simulink model "TV_FLC_codegen"  (R2025b)
settings: Solver=FixedStepDiscrete  StartTime=0.0  StopTime=100  FixedStep=0.003  MaxStep=0.4  RelTol=1e-3  AbsTol=1e-3
PreLoadFcn:
  | % Due to usability issue in Repeating Sequence block
  | warning('off','Simulink:Masking:Invalid');
  | 
  | % Eliminate unnecessary warnings in inactive variants
  | % Warnings generated only if you click through inactive variant
  | warning('off','MATLAB:nonExistentField');
  | warning('off','Simulink:Parameters:BlkParamUndefined');
PostLoadFcn:
  | set_param([bdroot '/Vehicle'],'popup_trailer','Off')
  | warning('off','sm:sli:setup:compile:LocalSolverNotSupported')
  | %sm_car_config_maneuver(bdroot,'WOT Braking');
  | sm_car_config_vehicle(bdroot,'false');
  | sm_car_config_logging(bdroot);
InitFcn:
  | sm_car_config_camera;
  | Vehicle = sm_car_vehcfg_checkConfig(Vehicle);
  | sm_car_check_tire_model(bdroot);
StartFcn:
  | tic;
StopFcn:
  | Elapsed_Sim_Time = toc;
  | % disp(['Elapsed Sim Time = ' num2str(Elapsed_Sim_Time)]);
model workspace (MAT data in the model file):
  Af = 1.20000004768
  C_alpha_F = 46504
  Control : object (value not decoded)
  F = 0.0421790704131
  FIS_1 : mamfis (value not decoded)
  FIS_2 : mamfis (value not decoded)
  FIS_3 : fistree (value not decoded)
  Gr = 5
  Ku = -0.000124337399029
  L = 1.57799994946
  Load_Ref = [0; 400; 500; 600; 700; 800; 900; 1000; 1100; 1200; 1300; 1400; 1500; 1600; 1700; 1800; 1900; 2000]
  MotorT = [51.0306892395 51.0306892395 51.0306892395 51.0306892395 51.0306892395 51.0306892395 51.0306892395 51.0306892395 51.0306892395 51.0306892395 51.0306892395 51.0306892395 51.0306892395 51.0306892395 51.0306892395 51.0306892395 51.0306892395 51.0306892395 51.0306892395 51.0306892395 51.0306892395 51.0306892395 51.0306892395 51.0306892395 51.0306892395 51.0306892395 51.0306892395 51.0306892395 51.0306892395 51.0306892395 51.0306892395 51.0306892395 51.0306892395 51.0306892395 51.0306892395 51.0306892395 51.0306892395 44.8436889648 36.8215675354 30.0627288818 25.3370742798 21.0374126434 17.0840320587 13.4184885025 9.99592685699 6.7769651413 3.73957490921]
  MotorW = [0 100 200 300 400 500 600 700 800 900 1000 1100 1200 1300 1400 1500 1600 1700 1800 1900 2000 2100 2200 2300 2400 2500 2600 2700 2800 2900 3000 3100 3200 3300 3400 3500 3600 3700 3800 3900 4000 4100 4200 4300 4400 4500 4600]
  Slip_Ctrl_Kd = Simulink.Parameter
  Slip_Ctrl_Kd.Value = 11
  Slip_Ctrl_Kd.Complexity = 'real'
  Slip_Ctrl_Kd.Dimensions = [1 1]
  Slip_Ctrl_Kd.CoderInfo.StorageClass = 'ImportedExtern'
  Slip_Ctrl_Kd.DataType = 'single'
  Slip_Ctrl_Ki = Simulink.Parameter
  Slip_Ctrl_Ki.Value = 6000
  Slip_Ctrl_Ki.Complexity = 'real'
  Slip_Ctrl_Ki.Dimensions = [1 1]
  Slip_Ctrl_Ki.CoderInfo.StorageClass = 'ImportedExtern'
  Slip_Ctrl_Ki.DataType = 'single'
  Slip_Ctrl_Kn = Simulink.Parameter
  Slip_Ctrl_Kn.Value = 100
  Slip_Ctrl_Kn.Complexity = 'real'
  Slip_Ctrl_Kn.Dimensions = [1 1]
  Slip_Ctrl_Kn.CoderInfo.StorageClass = 'ImportedExtern'
  Slip_Ctrl_Kn.DataType = 'single'
  Slip_Ctrl_Kp = Simulink.Parameter
  Slip_Ctrl_Kp.Value = 800
  Slip_Ctrl_Kp.Complexity = 'real'
  Slip_Ctrl_Kp.Dimensions = [1 1]
  Slip_Ctrl_Kp.CoderInfo.StorageClass = 'ImportedExtern'
  Slip_Ctrl_Kp.DataType = 'single'
  Slip_Ref = [0.0799999982119; 0.0799999982119; 0.0900000035763; 0.0949999988079; 0.0930000022054; 0.0920000001788; 0.0909999981523; 0.0900000035763; 0.0900000035763; 0.0900000035763; 0.0939999967813; 0.097999997437; 0.104000002146; 0.112000003457; 0.126000002027; 0.153999999166; 0.20000000298; 0.119999997318]
  Tmax = 51.0306892395
  a = 0.823199987411
  a_cop = 0.707000017166
  cd = -2.15000009537
  g = 9.81000041962
  h_CG = 0.358300000429
  m = 320
  ro = 1.22599995136
  rwheel = 0.263000011444
  steerRatio = 0.175131350756
  tr = 1.24800002575
  vx_th = 0.699999988079
libraries: simulink x5, fuzblock x3, slpidlib x2
(part 1 of 2)
settings Model: Creator=smiller  LastModifiedBy=andrei
settings SolverCC: MaxConsecutiveMinStep=5  AlgebraicLoopSolver=TrustRegion  AutoInsertRateTranBlk=on  InsertRTBMode=Never (minimum delay)  MinimalZcImpactIntegration=on
settings DataIOCC: MaxDataPoints=10000  SaveFormat=StructureWithTime  SaveOutput=off  SignalLogging=off  DSMLogging=off  SaveTime=off  ReturnWorkspaceOutputs=off  SignalLoggingName=logsout_sm_car
settings OptimizationCC: DefaultParameterBehavior=Inlined  UseDivisionForNetSlopeComputation=on  GainParamInheritBuiltInType=on  UseFloatMulNetSlope=on  DefaultUnderspecifiedDataType=single  UseSpecifiedMinMax=on  PassReuseOutputArgsAs=Individual arguments  NoFixptDivByZeroProtection=on  EfficientFloat2IntCast=on  LifeSpan=inf  OptimizeBlockOrder=speed  DifferentSizesBufferReuse=on  EfficientTunableParamExpr=on
settings DebuggingCC: ReadBeforeWriteMsg=EnableAllAsError  WriteAfterWriteMsg=EnableAllAsError  WriteAfterReadMsg=EnableAllAsError  AlgebraicLoopMsg=none  IntegerOverflowMsg=error  ParameterPrecisionLossMsg=none  ParameterTunabilityLossMsg=error  UnconnectedInputMsg=warning  UnconnectedOutputMsg=warning  UnconnectedLineMsg=warning  UniqueDataStoreMsg=error  NonBusSignalsTreatedAsBus=error  SFInvalidInputDataAccessInChartInitDiag=error  SFTransitionOutsideNaturalParentDiag=error  SFUnreachableExecutionPathDiag=error  SFUndirectedBroadcastEventsDiag=error  IntegerSaturationMsg=error  ArithmeticOperatorsInVariantConditions=warning
settings HardwareCC: ProdBitPerPointer=32.0  ProdBitPerSizeT=32.0  ProdBitPerPtrDiffT=32.0  ProdLargestAtomicInteger=Long  ProdLargestAtomicFloat=Double  ProdWordSize=32.0  ProdHWDeviceType=ARM Compatible->ARM Cortex-M
settings ModelReferenceCC: EnableRefExpFcnMdlSchedulingChecks=on
settings SFSimCC: MATLABDynamicMemAlloc=off  CustomCodeUndefinedFunction=UseInterfaceOnly
settings RTWCC: SystemTargetFile=ert.tlc  TemplateMakefile=ert_default_tmf  BuildConfiguration=Faster Runs  GPUComputeCapability=3.5  DLArmComputeVersion=19.05  Description=Embedded Coder
settings CodeAppCC: ForceParamTrailComments=on  IgnoreCustomStorageClasses=off  OperatorAnnotations=on  SimulinkDataObjDesc=on  SFDataObjDesc=on  CustomSymbolStrGlobalVar=rt$N_$R$M  CustomSymbolStrType=$N_$R$M  CustomSymbolStrFcn=$N$M$F  CustomSymbolStrMacro=$N$M  CustomSymbolStrUtil=$N_$R$C  InsertBlockDesc=on
settings ERTTargetCC: ERTCustomFileTemplate=example_file_process.tlc  ERTFilePackagingFormat=CompactWithDataFile  GenerateSampleERTMain=on  IncludeMdlTerminateFcn=off  CombineSignalStateStructs=on  SuppressErrorStatus=on  SupportAbsoluteTime=off  CodeInterfacePackaging=Reusable function  SupportComplex=off
settings SimscapeCC: SimscapeLogType=all  SimscapeLogSimulationStatistics=on  SimscapeLogName=simlog_sm_car  SimscapeLogDataHistory=100000.0  SimscapeOperatingPoint=ssc_op
settings DiagnosticsConfigSet: SimMechanicsConflictingReferenceFrames=none  SimMechanicsRigidlyBoundBlock=none  SimMechanicsUnsatisfiedHighPriorityTargets=error
settings ExplorerConfigSet: InternalSimMechanicsExplorerSettings="<ExplorerConfiguration><canonicalview>default</canonicalview><AnimationSetting><BasePlaybackSpeed>1.0</BasePlaybackSpeed><PlaybackSpeedFactor>1.0</PlaybackSpeedFactor></AnimationSetting><TilePanel><TileInfo><Tiles Columns=\"1\" Count=\"1\" Rows=\"1\"><Column Weight=\"1\"/><Row Weight=\"1\"/><Tile Height=\"1\" Width=\"1\" X=\"0\" Y=\"0\"/></Tiles></TileInfo><SceneInfo><SceneViewer><BGColor><R>1</R><G>1</G><B>1</B></BGColor><Camera><DoPerspective>on</DoPerspective><Position><X>-22.5734563329168161</X><Y>-2.56079992530625722</Y><Z>1.4393604008155032</Z></Position><Center><X>-23.2962680852000119</X><Y>-1.95845679840359432</Y><Z>1.10064823948317181</Z></Center><Up><X>-0.260205889993916473</X><Y>0.216838241661597014</Y><Z>0.940890042335224552</Z></Up><ViewLimDist>1</ViewLimDist><YLim>0.466307658154998694</YLim><XLim>0.489818968650208741</XLim></Camera></SceneViewer></SceneInfo></TilePanel><MechEditorPanel><Cameras><Camera><Id>Camera1</Id><Value><Name>Track FixO FR</Name><NativeCamera><PositionTrackingFeature>Camera_Frames.Frame_FixO_FR.R</PositionTrackingFeature><CenterTrackingFeature>Camera_Frames.Frame_FixO_FR.R</CenterTrackingFeature><UpVectorTrackingFeature>Camera_Frames.Frame_FixO_FR.R</UpVectorTrackingFeature><CenterTrackingOrigin>off</CenterTrackingOrigin><CenterTrackingDirection>+X</CenterTrackingDirection><UpVectorTrackingDirection>+Z</UpVectorTrackingDirection></NativeCamera></Value></Camera><Camera><Id>Camera2</Id><Value><Name>Track FixO Right</Name><NativeCamera><PositionTrackingFeature>Camera_Frames.Frame_FixO_Right.R</PositionTrackingFeature><CenterTrackingFeature>Camera_Frames.Transform_Camera_Ref.F</CenterTrackingFeature><UpVectorTrackingFeature>Camera_Frames.Frame_FixO_Right.R</UpVectorTrackingFeature><CenterTrackingOrigin>off</CenterTrackingOrigin><CenterTrackingDirection>+Y</CenterTrackingDirection><UpVectorTrackingDirection>+Z</UpVectorTrackingDirection></NativeCamera></Value></Camera><Camera><Id>Camera3</Id><Value><Name>Track FixO RR</Name><NativeCamera><PositionTrackingFeature>Camera_Frames.Frame_FixO_RR.R</PositionTrackingFeature><CenterTrackingFeature>Camera_Frames.Frame_FixO_RR.R</CenterTrackingFeature><UpVectorTrackingFeature>Camera_Frames.Frame_FixO_RR.R</UpVectorTrackingFeature><CenterTrackingOrigin>off</CenterTrackingOrigin><CenterTrackingDirection>+X</CenterTrackingDirection><UpVectorTrackingDirection>+Z</UpVectorTrackingDirection></NativeCamera></Value></Camera><Camera><Id>Camera4</Id><Value><Name>Track FixO RL</Name><NativeCamera><PositionTrackingFeature>Camera_Frames.Frame_FixO_RL.R</PositionTrackingFeature><CenterTrackingFeature>Camera_Frames.Frame_FixO_RL.R</CenterTrackingFeature><UpVectorTrackingFeature>Camera_Frames.Frame_FixO_RL.R</UpVectorTrackingFeature><CenterTrackingOrigin>off</CenterTrackingOrigin><CenterTrackingDirection>+X</CenterTrackingDirection><UpVectorTrackingDirection>+Z</UpVectorTrackingDirection></NativeCamera></Value></Camera><Camera><Id>Camera5</Id><Value><Name>Track FixO Left</Name><NativeCamera><PositionTrackingFeature>Camera_Frames.Frame_FixO_Left.R</PositionTrackingFeature><CenterTrackingFeature>Camera_Frames.Transform_Camera_Ref.F</CenterTrackingFeature><UpVectorTrackingFeature>Camera_Frames.Frame_FixO_Left.R</UpVectorTrackingFeature><CenterTrackingOrigin>off</CenterTrackingOrigin><CenterTrackingDirection>-Y</CenterTrackingDirection><UpVectorTrackingDirection>+Z</UpVectorTrackingDirection></NativeCamera></Value></Camera><Camera><Id>Camera6</Id><Value><Name>Track FixO FL</Name><NativeCamera><PositionTrackingFeature>Camera_Frames.Frame_FixO_FL.R</PositionTrackingFeature><CenterTrackingFeature>Camera_Frames.Frame_FixO_FL.R</CenterTrackingFeature><UpVectorTrackingFeature>Camera_Frames.Frame_FixO_FL.R</UpVectorTrackingFeature><CenterTrackingOrigin>off</CenterTrackingOrigin><CenterTrackingDirection>+X</CenterTrackingDirection><UpVectorTrackingDirection>+Z</UpVectorTrackingDirection></NativeCamera></Value></Camera><Camera><Id>Camera7</Id><Value><Name>Track FixO Top</Name><NativeCamera><PositionTrackingFeature>Camera_Frames.Frame_FixO_Top.R</PositionTrackingFeature><CenterTrackingFeature>Camera_Frames.Frame_FixO_Top.R</CenterTrackingFeature><UpVectorTrackingFeature>Camera_Frames.Frame_FixO_Top.R</UpVectorTrackingFeature><CenterTrackingOrigin>off</CenterTrackingOrigin><CenterTrackingDirection>+X</CenterTrackingDirection><UpVectorTrackingDirection>+Z</UpVectorTrackingDirection></NativeCamera></Value></Camera><Camera><Id>Camera8</Id><Value><Name>Track FixO Front</Name><NativeCamera><PositionTrackingFeature>Camera_Frames.Frame_FixO_Front.R</PositionTrackingFeature><CenterTrackingFeature>Camera_Frames.Frame_FixO_Front.R</CenterTrackingFeature><UpVectorTrackingFeature>Camera_Frames.Frame_FixO_Front.R</UpVectorTrackingFeature><CenterTrackingOrigin>off</CenterTrackingOrigin><CenterTrackingDirection>+X</CenterTrackingDirection><UpVectorTrackingDirection>+Z</UpVectorTrackingDirection></NativeCamera></Value></Camera><Camera><Id>Camera9</Id><Value><Name>Track FixO Rear</Name><NativeCamera><PositionTrackingFeature>Camera_Frames.Frame_FixO_Rear.R</PositionTrackingFeature><CenterTrackingFeature>Camera_Frames.Frame_FixO_Rear.R</CenterTrackingFeature><UpVectorTrackingFeature>Camera_Frames.Frame_FixO_Rear.R</UpVectorTrackingFeature><CenterTrackingOrigin>off</CenterTrackingOrigin><CenterTrackingDirection>+X</CenterTrackingDirection><UpVectorTrackingDirection>+Z</UpVectorTrackingDirection></NativeCamera></Value></Camera><Camera><Id>Camera10</Id><Value><Name>Track FR</Name><NativeCamera><PositionTrackingFeature>Camera_Frames.Frame_FR.R</PositionTrackingFeature><CenterTrackingFeature>Camera_Frames.Frame_FR.R</CenterTrackingFeature><UpVectorTrackingFeature>Camera_Frames.Frame_FR.R</UpVectorTrackingFeature><CenterTrackingOrigin>off</CenterTrackingOrigin><CenterTrackingDirection>+X</CenterTrackingDirection><UpVectorTrackingDirection>+Z</UpVectorTrackingDirection></NativeCamera></Value></Camera><Camera><Id>Camera11</Id><Value><Name>Track Right</Name><NativeCamera><PositionTrackingFeature>Camera_Frames.Frame_Right.R</PositionTrackingFeature><CenterTrackingFeature>Camera_Frames.Transform_Camera_Ref.F</CenterTrackingFeature><UpVectorTrackingFeature>Camera_Frames.Frame_Right.R</UpVectorTrackingFeature><CenterTrackingOrigin>off</CenterTrackingOrigin><CenterTrackingDirection>+Y</CenterTrackingDirection><UpVectorTrackingDirection>+Z</UpVectorTrackingDirection></NativeCamera></Value></Camera><Camera><Id>Camera12</Id><Value><Name>Track RR</Name><NativeCamera><PositionTrackingFeature>Camera_Frames.Frame_RR.R</PositionTrackingFeature><CenterTrackingFeature>Camera_Frames.Frame_RR.R</CenterTrackingFeature><UpVectorTrackingFeature>Camera_Frames.Frame_RR.R</UpVectorTrackingFeature><CenterTrackingOrigin>off</CenterTrackingOrigin><CenterTrackingDirection>+X</CenterTrackingDirection><UpVectorTrackingDirection>+Z</UpVectorTrackingDirection></NativeCamera></Value></Camera><Camera><Id>Camera13</Id><Value><Name>Track RL</Name><NativeCamera><PositionTrackingFeature>Camera_Frames.Frame_RL.R</PositionTrackingFeature><CenterTrackingFeature>Camera_Frames.Frame_RL.R</CenterTrackingFeature><UpVectorTrackingFeature>Camera_Frames.Frame_RL.R</UpVectorTrackingFeature><CenterTrackingOrigin>off</CenterTrackingOrigin><CenterTrackingDirection>+X</CenterTrackingDirection><UpVectorTrackingDirection>+Z</UpVectorTrackingDirection></NativeCamera></Value></Camera><Camera><Id>Camera14</Id><Value><Name>Track Left</Name><NativeCamera><PositionTrackingFeature>Camera_Frames.Frame_Left.R</PositionTrackingFeature><CenterTrackingFeature>Camera_Frames.Transform_Camera_Ref.F</CenterTrackingFeature><UpVectorTrackingFeature>Camera_Frames.Frame_Left.R</UpVectorTrackingFeature><CenterTrackingOrigin>off</CenterTrackingOrigin><CenterTrackingDirection>-Y</CenterTrackingDirection><UpVectorTrackingDirection>+Z</UpVectorTrackingDirection></NativeCamera></Value></Camera><Camera><Id>Camera15</Id><Value><Name>Track FL</Name><NativeCamera><PositionTrackingFeature>Camera_Frames.Frame_FL.R</PositionTrackingFeature><CenterTrackingFeature>Camera_Frames.Frame_FL.R</CenterTrackingFeature><UpVectorTrackingFeature>Camera_Frames.Frame_FL.R</UpVectorTrackingFeature><CenterTrackingOrigin>off</CenterTrackingOrigin><CenterTrackingDirection>+X</CenterTrackingDirection><UpVectorTrackingDirection>+Z</UpVectorTrackingDirection></NativeCamera></Value></Camera><Camera><Id>Camera16</Id><Value><Name>Track Top</Name><NativeCamera><PositionTrackingFeature>Camera_Frames.Frame_Top.R</PositionTrackingFeature><CenterTrackingFeature>Camera_Frames.Frame_Top.R</CenterTrackingFeature><UpVectorTrackingFeature>Camera_Frames.Frame_Top.R</UpVectorTrackingFeature><CenterTrackingOrigin>off</CenterTrackingOrigin><CenterTrackingDirection>+X</CenterTrackingDirection><UpVectorTrackingDirection>+Z</UpVectorTrackingDirection></NativeCamera></Value></Camera><Camera><Id>Camera17</Id><Value><Name>Track Front</Name><NativeCamera><PositionTrackingFeature>Camera_Frames.Frame_Front.R</PositionTrackingFeature><CenterTrackingFeature>Camera_Frames.Frame_Front.R</CenterTrackingFeature><UpVectorTrackingFeature>Camera_Frames.Frame_Front.R</UpVectorTrackingFeature><CenterTrackingOrigin>off</CenterTrackingOrigin><CenterTrackingDirection>+X</CenterTrackingDirection><UpVectorTrackingDirection>+Z</UpVectorTrackingDirection></NativeCamera></Value></Camera><Camera><Id>Camera18</Id><Value><Name>Track Rear</Name><NativeCamera><PositionTrackingFeature>Camera_Frames.Frame_Rear.R</PositionTrackingFeature><CenterTrackingFeature>Camera_Frames.Frame_Rear.R</CenterTrackingFeature><UpVectorTrackingFeature>Camera_Frames.Frame_Rear.R</UpVectorTrackingFeature><CenterTrackingOrigin>off</CenterTrackingOrigin><CenterTrackingDirection>+X</CenterTrackingDirection><UpVectorTrackingDirection>+Z</UpVectorTrackingDirection></NativeCamera></Value></Camera><Camera><Id>Camera19</Id><Value><Name>Track SuspF</Name><NativeCamera><PositionTrackingFeature>Camera_Frames.Frame_SuspF.R</PositionTrackingFeature><CenterTrackingFeature>Camera_Frames.Frame_SuspF.R</CenterTrackingFeature><UpVectorTrackingFeature>Camera_Frames.Frame_SuspF.R</UpVectorTrackingFeature><CenterTrackingOrigin>off</CenterTrackingOrigin><CenterTrackingDirection>+X</CenterTrackingDirection><UpVectorTrackingDirection>+Z</UpVectorTrackingDirection></NativeCamera></Value></Camera><Camera><Id>Camera20</Id><Value><Name>Track SuspR</Name><NativeCamera><PositionTrackingFeature>Camera_Frames.Frame_SuspR.R</PositionTrackingFeature><CenterTrackingFeature>Camera_Frames.Frame_SuspR.R</CenterTrackingFeature><UpVectorTrackingFeature>Camera_Frames.Frame_SuspR.R</UpVectorTrackingFeature><CenterTrackingOrigin>off</CenterTrackingOrigin><CenterTrackingDirection>+X</CenterTrackingDirection><UpVectorTrackingDirection>+Z</UpVectorTrackingDirection></NativeCamera></Value></Camera><Camera><Id>Camera21</Id><Value><Name>Track WheelFR</Name><NativeCamera><PositionTrackingFeature>Camera_Frames.Frame_Wheel_FR.R</PositionTrackingFeature><CenterTrackingFeature>Camera_Frames.Frame_Wheel_FR.R</CenterTrackingFeature><UpVectorTrackingFeature>Camera_Frames.Frame_Wheel_FR.R</UpVectorTrackingFeature><CenterTrackingOrigin>off</CenterTrackingOrigin><CenterTrackingDirection>+X</CenterTrackingDirection><UpVectorTrackingDirection>+Z</UpVectorTrackingDirection></NativeCamera></Value></Camera><Camera><Id>Camera22</Id><Value><Name>Track WheelRR</Name><NativeCamera><PositionTrackingFeature>Camera_Frames.Frame_Wheel_RR.R</PositionTrackingFeature><CenterTrackingFeature>Camera_Frames.Frame_Wheel_RR.R</CenterTrackingFeature><UpVectorTrackingFeature>Camera_Frames.Frame_Wheel_RR.R</UpVectorTrackingFeature><CenterTrackingOrigin>off</CenterTrackingOrigin><CenterTrackingDirection>+X</CenterTrackingDirection><UpVectorTrackingDirection>+Z</UpVectorTrackingDirection></NativeCamera></Value></Camera><Camera><Id>Camera23</Id><Value><Name>Track WheelRL</Name><NativeCamera><PositionTrackingFeature>Camera_Frames.Frame_Wheel_RL.R</PositionTrackingFeature><CenterTrackingFeature>Camera_Frames.Frame_Wheel_RL.R</CenterTrackingFeature><UpVectorTrackingFeature>Camera_Frames.Frame_Wheel_RL.R</UpVectorTrackingFeature><CenterTrackingOrigin>off</CenterTrackingOrigin><CenterTrackingDirection>+X</CenterTrackingDirection><UpVectorTrackingDirection>+Z</UpVectorTrackingDirection></NativeCamera></Value></Camera><Camera><Id>Camera24</Id><Value><Name>Track WheelFL</Name><NativeCamera><PositionTrackingFeature>Camera_Frames.Frame_Wheel_FL.R</PositionTrackingFeature><CenterTrackingFeature>Camera_Frames.Frame_Wheel_FL.R</CenterTrackingFeature><UpVectorTrackingFeature>Camera_Frames.Frame_Wheel_FL.R</UpVectorTrackingFeature><CenterTrackingOrigin>off</CenterTrackingOrigin><CenterTrackingDirection>+X</CenterTrackingDirection><UpVectorTrackingDirection>+Z</UpVectorTrackingDirection></NativeCamera></Value></Camera><Camera><Id>Camera25</Id><Value><Name>View Seat FL</Name><NativeCamera><PositionTrackingFeature>Camera_Frames.Frame_View_Seat_FL.R</PositionTrackingFeature><CenterTrackingFeature>Camera_Frames.Frame_View_Seat_FL.R</CenterTrackingFeature><UpVectorTrackingFeature>Camera_Frames.Frame_View_Seat_FL.R</UpVectorTrackingFeature><CenterTrackingOrigin>off</CenterTrackingOrigin><CenterTrackingDirection>+X</CenterTrackingDirection><UpVectorTrackingDirection>+Z</UpVectorTrackingDirection></NativeCamera></Value></Camera><Camera><Id>Camera26</Id><Value><Name>View Seat FR</Name><NativeCamera><PositionTrackingFeature>Camera_Frames.Frame_View_Seat_FR.R</PositionTrackingFeature><CenterTrackingFeature>Camera_Frames.Frame_View_Seat_FR.R</CenterTrackingFeature><UpVectorTrackingFeature>Camera_Frames.Frame_View_Seat_FR.R</UpVectorTrackingFeature><CenterTrackingOrigin>off</CenterTrackingOrigin><CenterTrackingDirection>+X</CenterTrackingDirection><UpVectorTrackingDirection>+Z</UpVectorTrackingDirection></NativeCamera></Value></Camera><Camera><Id>Camera27</Id><Value><Name>View Susp FR</Name><NativeCamera><PositionTrackingFeature>Camera_Frames.Frame_View_Susp_FR.R</PositionTrackingFeature><CenterTrackingFeature>Camera_Frames.Frame_View_Susp_FR.R</CenterTrackingFeature><UpVectorTrackingFeature>Camera_Frames.Frame_View_Susp_FR.R</UpVectorTrackingFeature><CenterTrackingOrigin>off</CenterTrackingOrigin><CenterTrackingDirection>+X</CenterTrackingDirection><UpVectorTrackingDirection>+Z</UpVectorTrackingDirection></NativeCamera></Value></Camera><Camera><Id>Camera28</Id><Value><Name>View Susp RR</Name><NativeCamera><PositionTrackingFeature>Camera_Frames.Frame_View_Susp_RR.R</PositionTrackingFeature><CenterTrackingFeature>Camera_Frames.Frame_View_Susp_RR.R</CenterTrackingFeature><UpVectorTrackingFeature>Camera_Frames.Frame_View_Susp_RR.R</UpVectorTrackingFeature><CenterTrackingOrigin>off</CenterTrackingOrigin><CenterTrackingDirection>+X</CenterTrackingDirection><UpVectorTrackingDirection>+Z</UpVectorTrackingDirection></NativeCamera></Value></Camera><Camera><Id>Camera29</Id><Value><Name>View Susp RL</Name><NativeCamera><PositionTrackingFeature>Camera_Frames.Frame_View_Susp_RL.R</PositionTrackingFeature><CenterTrackingFeature>Camera_Frames.Frame_View_Susp_RL.R</CenterTrackingFeature><UpVectorTrackingFeature>Camera_Frames.Frame_View_Susp_RL.R</UpVectorTrackingFeature><CenterTrackingOrigin>off</CenterTrackingOrigin><CenterTrackingDirection>+X</CenterTrackingDirection><UpVectorTrackingDirection>+Z</UpVectorTrackingDirection></NativeCamera></Value></Camera><Camera><Id>Camera30</Id><Value><Name>View Susp FL</Name><NativeCamera><PositionTrackingFeature>Camera_Frames.Frame_View_Susp_FL.R</PositionTrackingFeature><CenterTrackingFeature>Camera_Frames.Frame_View_Susp_FL.R</CenterTrackingFeature><UpVectorTrackingFeature>Camera_Frames.Frame_View_Susp_FL.R</UpVectorTrackingFeature><CenterTrackingOrigin>off</CenterTrackingOrigin><CenterTrackingDirection>+X</CenterTrackingDirection><UpVectorTrackingDirection>+Z</UpVectorTrackingDirection></NativeCamera></Value></Camera><Camera><Id>Camera31</Id><Value><Name>Dolly Camera</Name><NativeCamera><PositionTrackingFeature>Camera_Frames.Frame_Dolly.R</PositionTrackingFeature><CenterTrackingFeature>Camera_Frames.Frame_Dolly.R</CenterTrackingFeature><UpVectorTrackingFeature>Camera_Frames.Frame_Dolly.R</UpVectorTrackingFeature><CenterTrackingOrigin>off</CenterTrackingOrigin><CenterTrackingDirection>+X</CenterTrackingDirection><UpVectorTrackingDirection>+Z</UpVectorTrackingDirection></NativeCamera></Value></Camera><Camera><Id>Camera32</Id><Value><Name>Track Dolly Camera</Name><NativeCamera><PositionTrackingFeature>Camera_Frames.Frame_Dolly.R</PositionTrackingFeature><CenterTrackingFeature>Camera_Frames.Transform_Camera_Ref.F</CenterTrackingFeature><UpVectorTrackingFeature>Camera_Frames.World_Frame.W</UpVectorTrackingFeature><CenterTrackingOrigin>on</CenterTrackingOrigin><UpVectorTrackingDirection>+Z</UpVectorTrackingDirection></NativeCamera></Value></Camera></Cameras><GfxPanelCameraMap><MapElement CameraMLId=\"Camera1\" GfxPanelIndex=\"0\"/></GfxPanelCameraMap><VideoCreator><PlaybackSpeedRatio>1.0</PlaybackSpeedRatio><FrameRate>30</FrameRate><VideoFormat>MPEG-4</VideoFormat><FrameSize>[800 450]</FrameSize></VideoCreator></MechEditorPanel></ExplorerConfiguration>"

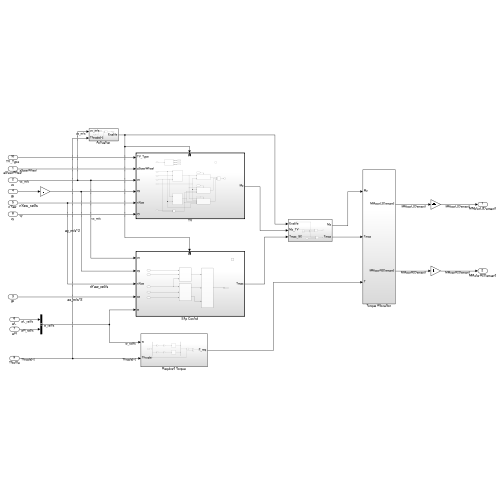
[thumbnail: Simulink's stored preview of the top-level diagram]
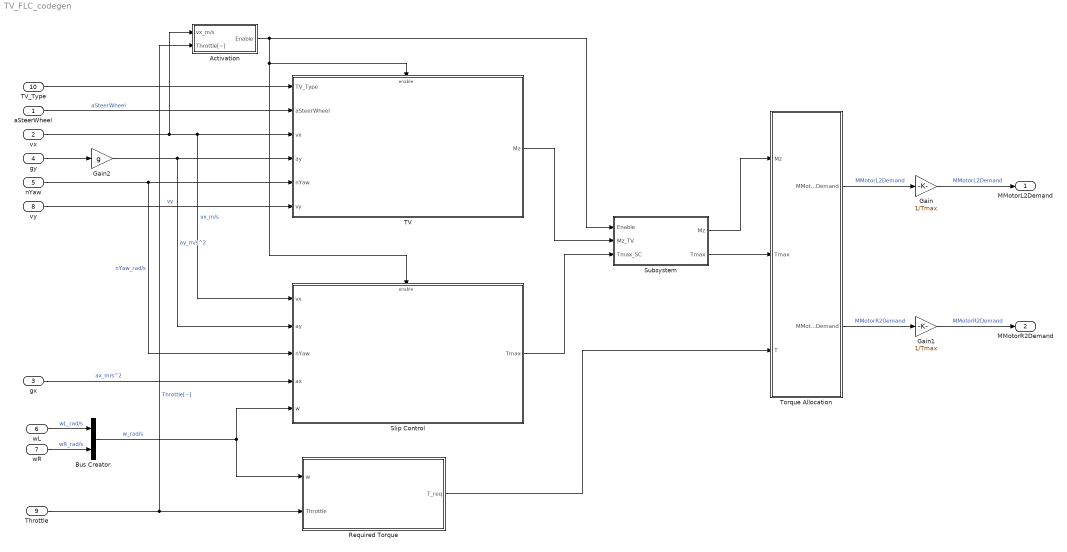
== system TV_FLC_codegen ==
  aSteerWheel : Inport  OutDataTypeStr=single  PortDimensions=1  SampleTime=0.003
  vx : Inport  Port=2  OutDataTypeStr=single  PortDimensions=1  SampleTime=0.003
  gx : Inport  Port=3  OutDataTypeStr=single  PortDimensions=1  SampleTime=0.003
  gy : Inport  Port=4  OutDataTypeStr=single  PortDimensions=1  SampleTime=0.003
  nYaw : Inport  Port=5  OutDataTypeStr=single  PortDimensions=1  SampleTime=0.003
  wL : Inport  Port=6  OutDataTypeStr=single  PortDimensions=1  SampleTime=0.003
  wR : Inport  Port=7  OutDataTypeStr=single  PortDimensions=1  SampleTime=0.003
  vy : Inport  Port=8  OutDataTypeStr=single  PortDimensions=1  SampleTime=0.003
  Throttle : Inport  Port=9  OutDataTypeStr=single  PortDimensions=1  SampleTime=0.003
  TV_Type : Inport  Port=10  OutDataTypeStr=single  PortDimensions=1  SampleTime=0.003
  Activation : Subsystem
  Bus Creator : BusCreator  Inputs=2
  Gain : Gain  Gain=1/Tmax  ParamDataTypeStr=single  OutDataTypeStr=single
  Gain1 : Gain  Gain=1/Tmax  ParamDataTypeStr=single  OutDataTypeStr=single
  Gain2 : Gain  Gain=g
  Required Torque : Subsystem
  Slip Control : Subsystem
  Subsystem : Subsystem
  TV : Subsystem
  Torque Allocation : Subsystem
  MMotorL2Demand : Outport  OutDataTypeStr=single  PortDimensions=1  SampleTime=0.003
  MMotorR2Demand : Outport  Port=2  OutDataTypeStr=single  PortDimensions=1  SampleTime=0.003
  wires:
  Torque Allocation/1(MMotorL2Demand) -> Gain/1  "MMotorL2Demand"
  wL/1 -> Bus Creator/1  "wL_rad/s"
  gy/1 -> Gain2/1
  Gain1/1 -> MMotorR2Demand/1  "MMotorR2Demand"
  Gain/1 -> MMotorL2Demand/1  "MMotorL2Demand"
  Torque Allocation/2(MMotorR2Demand) -> Gain1/1  "MMotorR2Demand"
  wR/1 -> Bus Creator/2  "wR_rad/s"
  Slip Control/1(Tmax) -> Subsystem/3(Tmax_SC)
  Required Torque/1(T_req) -> Torque Allocation/3(T)
  aSteerWheel/1 -> TV/2(aSteerWheel)  "aSteerWheel"
  Gain2/1 -> TV/4(ay), Slip Control/2(ay)  "ay_m/s^2"
  Bus Creator/1 -> Slip Control/5(w), Required Torque/1(w)  "w_rad/s"
  nYaw/1 -> TV/5(nYaw), Slip Control/3(nYaw)  "nYaw_rad/s"
  gx/1 -> Slip Control/4(ax)  "ax_m/s^2"
  Throttle/1 -> Activation/2(Throttle[~]), Required Torque/2(Throttle)  "Throttle[~]"
  TV/1(Mz) -> Subsystem/2(Mz_TV)
  vy/1 -> TV/6(vy)  "vy"
  vx/1 -> TV/3(vx), Slip Control/1(vx), Activation/1(vx_m/s)  "vx_m/s"
  Activation/1(Enable) -> Slip Control/Enable, TV/Enable, Subsystem/1(Enable)
  Subsystem/1(Mz) -> Torque Allocation/1(Mz)
  Subsystem/2(Tmax) -> Torque Allocation/2(Tmax)
  TV_Type/1 -> TV/1(TV_Type)

== system TV_FLC_codegen/Activation ==
  vx_m/s : Inport
  Throttle[~] : Inport  Port=2
  AND : Logic  AllPortsSameDT=off  OutDataTypeStr=boolean
  Compare To Zero : simulink/Logic and Bit Operations/Compare To Zero  relop=~=  OutDataTypeStr=boolean
  Relational Operator : RelationalOperator  Operator=<=  OutDataTypeStr=boolean  RndMeth=Simplest  InputSameDT=off
  th_vx_min : Constant  Value=vx_th
  Enable : Outport
  wires:
  Compare To Zero/1 -> AND/2
  AND/1 -> Enable/1
  Throttle[~]/1 -> Compare To Zero/1
  th_vx_min/1 -> Relational Operator/1
  vx_m/s/1 -> Relational Operator/2
  Relational Operator/1 -> AND/1

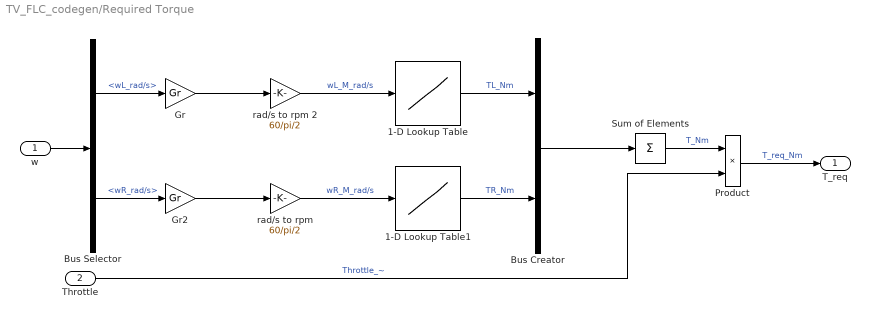
== system TV_FLC_codegen/Required Torque ==
  w : Inport
  Throttle : Inport  Port=2
  1-D Lookup Table : Lookup_n-D  NumberOfTableDimensions=1  BreakpointsForDimension1=MotorW  Table=MotorT  InternalRulePriority=Speed  RndMeth=Simplest
  1-D Lookup Table1 : Lookup_n-D  NumberOfTableDimensions=1  BreakpointsForDimension1=MotorW  Table=MotorT  InternalRulePriority=Speed  RndMeth=Simplest
  Bus Creator : BusCreator  Inputs=2
  Bus Selector : BusSelector  OutputSignals=wL_rad/s,wR_rad/s
  Gr : Gain  Gain=Gr
  Gr2 : Gain  Gain=Gr
  Product : Product
  Sum of Elements : Sum  Inputs=+
  rad/s to rpm : Gain  Gain=60/pi/2
  rad/s to rpm 2 : Gain  Gain=60/pi/2
  T_req : Outport
  wires:
  Gr2/1 -> rad/s to rpm/1
  Gr/1 -> rad/s to rpm 2/1
  Bus Creator/1 -> Sum of Elements/1
  1-D Lookup Table/1 -> Bus Creator/1  "TL_Nm"
  rad/s to rpm 2/1 -> 1-D Lookup Table/1  "wL_M_rad/s"
  Bus Selector/2 -> Gr2/1  "<wR_rad/s>"
  Product/1 -> T_req/1  "T_req_Nm"
  Bus Selector/1 -> Gr/1  "<wL_rad/s>"
  rad/s to rpm/1 -> 1-D Lookup Table1/1  "wR_M_rad/s"
  Throttle/1 -> Product/2  "Throttle_~"
  1-D Lookup Table1/1 -> Bus Creator/2  "TR_Nm"
  Sum of Elements/1 -> Product/1  "T_Nm"
  w/1 -> Bus Selector/1

== system TV_FLC_codegen/Slip Control ==
  vx : Inport
  ay : Inport  Port=2
  nYaw : Inport  Port=3
  ax : Inport  Port=4
  w : Inport  Port=5
  Enable : EnablePort  StatesWhenEnabling=reset
  Loads : Subsystem
  Maximum Torque Allowed : Subsystem
  Slip Calculation : Subsystem
  Tmax : Outport
  wires:
  w/1 -> Slip Calculation/3(w)  "w_rad/s"
  nYaw/1 -> Slip Calculation/2(nYaw)  "nYaw_rad/s"
  ax/1 -> Loads/1(ax)  "ax_m/s^2"
  Loads/1(Fz) -> Maximum Torque Allowed/1(Fz)
  ay/1 -> Loads/2(ay)  "ay_m/s^2"
  Slip Calculation/2(kappa_rr) -> Maximum Torque Allowed/3(kappa_rr)
  vx/1 -> Loads/3(vx), Slip Calculation/1(Vx)  "vx_m/s"
  Maximum Torque Allowed/1(Tmax) -> Tmax/1
  Slip Calculation/1(kappa_rl) -> Maximum Torque Allowed/2(kappa_rl)

== system TV_FLC_codegen/Subsystem ==
  Enable : Inport
  Mz_TV : Inport  Port=2
  Tmax_SC : Inport  Port=3
  Bus Creator1 : BusCreator  Inputs=2
  Constant : Constant  Value=Tmax
  Constant1 : Constant  Value=Tmax
  Constant2 : Constant  Value=0
  Switch : Switch  Criteria=u2 ~= 0  SaturateOnIntegerOverflow=off  InputSameDT=off
  Switch1 : Switch  Criteria=u2 ~= 0  SaturateOnIntegerOverflow=off  InputSameDT=off
  Mz : Outport
  Tmax : Outport  Port=2
  wires:
  Switch1/1 -> Mz/1
  Constant2/1 -> Switch1/3  "Mz"
  Mz_TV/1 -> Switch1/1
  Constant/1 -> Bus Creator1/1  "Tmax_rl_Nm"
  Tmax_SC/1 -> Switch/1
  Bus Creator1/1 -> Switch/3
  Switch/1 -> Tmax/1
  Constant1/1 -> Bus Creator1/2  "Tmax_rr_Nm"
  Enable/1 -> Switch/2, Switch1/2

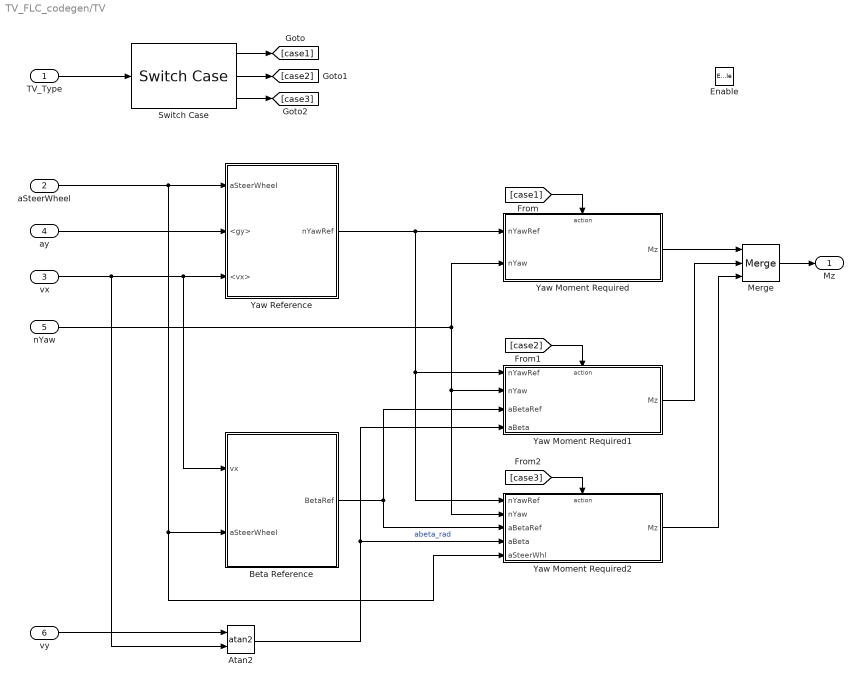
== system TV_FLC_codegen/TV ==
  TV_Type : Inport
  aSteerWheel : Inport  Port=2
  vx : Inport  Port=3
  ay : Inport  Port=4
  nYaw : Inport  Port=5
  vy : Inport  Port=6
  Enable : EnablePort  StatesWhenEnabling=reset
  Atan2 : Trigonometry  Operator=atan2
  Beta Reference : Subsystem
  Merge : Merge  Inputs=3
  Switch Case : SwitchCase  CaseConditions={1, 2, 3}  ShowDefaultCase=off
  Yaw Moment Required : Subsystem
  Yaw Moment Required1 : Subsystem
  Yaw Moment Required2 : Subsystem
  Yaw Reference : Subsystem
  Mz : Outport
  wires:
  Merge/1 -> Mz/1
  Yaw Moment Required2/1(Mz) -> Merge/3
  [case3] -> Yaw Moment Required2/Action
  Switch Case/3 -> [case3]
  [case2] -> Yaw Moment Required1/Action
  Switch Case/2 -> [case2]
  [case1] -> Yaw Moment Required/Action
  Switch Case/1 -> [case1]
  Atan2/1 -> Yaw Moment Required2/4(aBeta), Yaw Moment Required1/4(aBeta)  "abeta_rad"
  Yaw Moment Required1/1(Mz) -> Merge/2
  TV_Type/1 -> Switch Case/1
  aSteerWheel/1 -> Yaw Moment Required2/5(aSteerWhl), Beta Reference/2(aSteerWheel), Yaw Reference/1(aSteerWheel)
  vx/1 -> Yaw Reference/3(<vx>), Beta Reference/1(vx), Atan2/2
  nYaw/1 -> Yaw Moment Required1/2(nYaw), Yaw Moment Required2/2(nYaw), Yaw Moment Required/2(nYaw)
  ay/1 -> Yaw Reference/2(<gy>)
  Yaw Moment Required/1(Mz) -> Merge/1
  Yaw Reference/1(nYawRef) -> Yaw Moment Required1/1(nYawRef), Yaw Moment Required2/1(nYawRef), Yaw Moment Required/1(nYawRef)
  Beta Reference/1(BetaRef) -> Yaw Moment Required2/3(aBetaRef), Yaw Moment Required1/3(aBetaRef)
  vy/1 -> Atan2/1

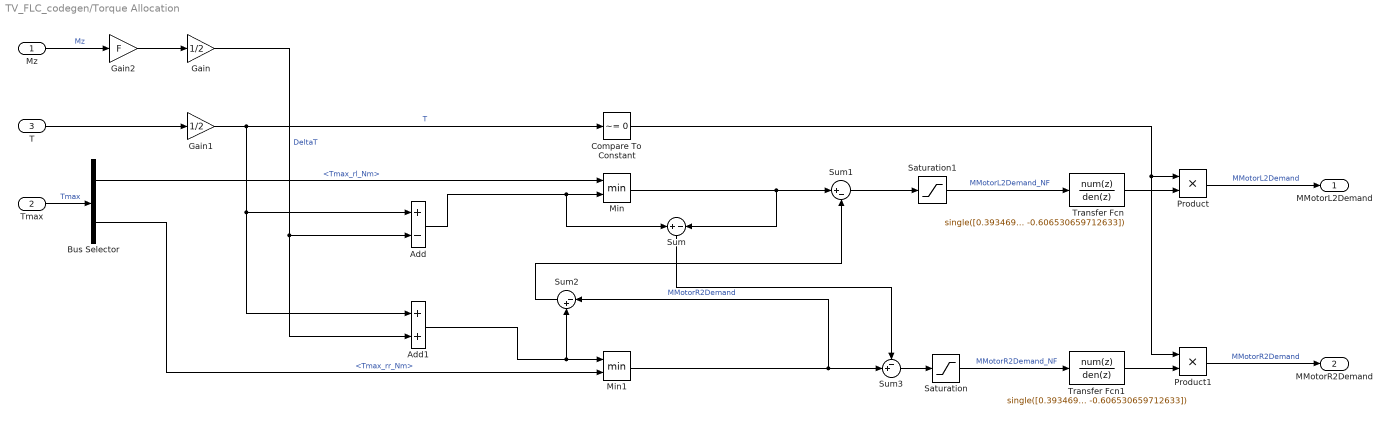
== system TV_FLC_codegen/Torque Allocation ==
  Mz : Inport  OutDataTypeStr=single
  Tmax : Inport  Port=2  OutDataTypeStr=single
  T : Inport  Port=3  OutDataTypeStr=single
  Add : Sum  Inputs=+-  OutDataTypeStr=single  AccumDataTypeStr=single
  Add1 : Sum  OutDataTypeStr=single  AccumDataTypeStr=single
  Bus Selector : BusSelector  OutputSignals=Tmax_rl_Nm,Tmax_rr_Nm
  Compare To Constant : simulink/Logic and Bit Operations/Compare To Constant  relop=~=  const=0  OutDataTypeStr=boolean
  Gain : Gain  Gain=1/2  ParamDataTypeStr=single  OutDataTypeStr=single
  Gain1 : Gain  Gain=1/2  ParamDataTypeStr=single  OutDataTypeStr=single
  Gain2 : Gain  Gain=F  ParamDataTypeStr=single  OutDataTypeStr=single
  Min : MinMax  Inputs=2  OutDataTypeStr=single
  Min1 : MinMax  Inputs=2  OutDataTypeStr=single
  Product : Product  OutDataTypeStr=single
  Product1 : Product  OutDataTypeStr=single
  Saturation : Saturate  UpperLimit=Tmax  LowerLimit=0  OutDataTypeStr=single
  Saturation1 : Saturate  UpperLimit=Tmax  LowerLimit=0  OutDataTypeStr=single
  Sum : Sum  Inputs=+|-  OutDataTypeStr=single  AccumDataTypeStr=single
  Sum1 : Sum  Inputs=|+-  OutDataTypeStr=single  AccumDataTypeStr=single
  Sum2 : Sum  Inputs=|-+  OutDataTypeStr=single  AccumDataTypeStr=single
  Sum3 : Sum  Inputs=-+|  OutDataTypeStr=single  AccumDataTypeStr=single
  Transfer Fcn : DiscreteTransferFcn  Numerator=single([0.393469340287367])  Denominator=single([1 -0.606530659712633])  SampleTime=0.003
  Transfer Fcn1 : DiscreteTransferFcn  Numerator=single([0.393469340287367])  Denominator=single([1 -0.606530659712633])  SampleTime=0.003
  MMotorL2Demand : Outport  OutDataTypeStr=single
  MMotorR2Demand : Outport  Port=2  OutDataTypeStr=single
  wires:
  Sum3/1 -> Saturation/1
  Sum1/1 -> Saturation1/1
  Gain2/1 -> Gain/1
  Gain/1 -> Add1/2, Add/2  "DeltaT"
  T/1 -> Gain1/1
  Mz/1 -> Gain2/1  "Mz"
  Min/1 -> Sum1/1, Sum/2
  Min1/1 -> Sum2/1, Sum3/2  "MMotorR2Demand"
  Tmax/1 -> Bus Selector/1  "Tmax"
  Bus Selector/1 -> Min/1  "<Tmax_rl_Nm>"
  Bus Selector/2 -> Min1/2  "<Tmax_rr_Nm>"
  Add/1 -> Sum/1, Min/2
  Add1/1 -> Sum2/2, Min1/1
  Sum2/1 -> Sum1/2
  Sum/1 -> Sum3/1
  Gain1/1 -> Compare To Constant/1, Add1/1, Add/1  "T"
  Compare To Constant/1 -> Product/1, Product1/1
  Product/1 -> MMotorL2Demand/1  "MMotorL2Demand"
  Product1/1 -> MMotorR2Demand/1  "MMotorR2Demand"
  Saturation1/1 -> Transfer Fcn/1  "MMotorL2Demand_NF"
  Transfer Fcn/1 -> Product/2
  Saturation/1 -> Transfer Fcn1/1  "MMotorR2Demand_NF"
  Transfer Fcn1/1 -> Product1/2

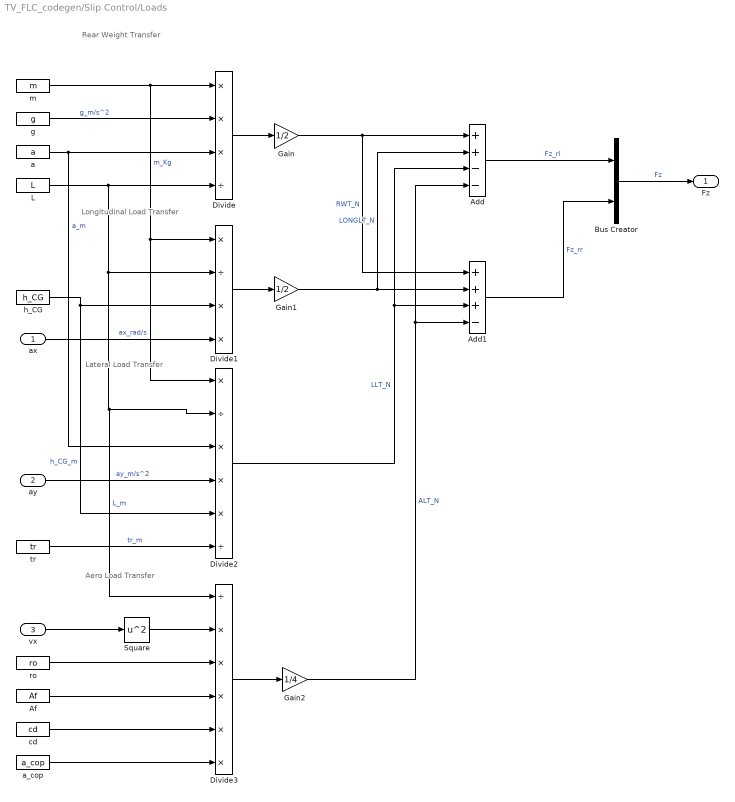
== system TV_FLC_codegen/Slip Control/Loads ==
  note: Aero Load Transfer
  note: Lateral Load Transfer
  note: Longitudinal Load Transfer
  note: Rear Weight Transfer
  ax : Inport
  ay : Inport  Port=2
  vx : Inport  Port=3
  Add : Sum  Inputs=++--
  Add1 : Sum  Inputs=+++-
  Af : Constant  Value=Af
  Bus Creator : BusCreator  Inputs=2
  Divide : Product  Inputs=***/
  Divide1 : Product  Inputs=*/**
  Divide2 : Product  Inputs=*/***/
  Divide3 : Product  Inputs=/*****
  Gain : Gain  Gain=1/2
  Gain1 : Gain  Gain=1/2
  Gain2 : Gain  Gain=1/4
  L : Constant  Value=L
  Square : Math  Operator=square
  a : Constant  Value=a
  a_cop : Constant  Value=a_cop
  cd : Constant  Value=cd
  g : Constant  Value=g
  h_CG : Constant  Value=h_CG
  m : Constant  Value=m
  ro : Constant  Value=ro
  tr : Constant  Value=tr
  Fz : Outport
  wires:
  m/1 -> Divide/1, Divide1/1, Divide2/1  "m_Kg"
  g/1 -> Divide/2  "g_m/s^2"
  a/1 -> Divide/3, Divide2/3  "a_m"
  L/1 -> Divide3/1, Divide2/2, Divide1/2, Divide/4  "L_m"
  Divide/1 -> Gain/1
  vx/1 -> Square/1
  Square/1 -> Divide3/2
  Gain/1 -> Add/1, Add1/1  "RWT_N"
  Gain2/1 -> Add/4, Add1/4  "ALT_N"
  h_CG/1 -> Divide2/5, Divide1/3  "h_CG_m"
  ax/1 -> Divide1/4  "ax_rad/s"
  Divide1/1 -> Gain1/1
  Gain1/1 -> Add/2, Add1/2  "LONGLT_N"
  ay/1 -> Divide2/4  "ay_m/s^2"
  tr/1 -> Divide2/6  "tr_m"
  Divide2/1 -> Add/3, Add1/3  "LLT_N"
  Add/1 -> Bus Creator/1  "Fz_rl"
  Add1/1 -> Bus Creator/2  "Fz_rr"
  Bus Creator/1 -> Fz/1  "Fz"
  Divide3/1 -> Gain2/1
  ro/1 -> Divide3/3
  Af/1 -> Divide3/4
  cd/1 -> Divide3/5
  a_cop/1 -> Divide3/6

== system TV_FLC_codegen/Slip Control/Maximum Torque Allowed ==
  Fz : Inport
  kappa_rl : Inport  Port=2
  kappa_rr : Inport  Port=3
  Bus Creator : BusCreator  Inputs=2
  Bus Selector : BusSelector  OutputSignals=Fz_rl,Fz_rr
  Slip Correction Left : Subsystem
  Slip Correction Right : Subsystem
  Tmax : Outport
  wires:
  Slip Correction Right/1(Tmax_rr) -> Bus Creator/2  "Tmax_rr_Nm"
  Slip Correction Left/1(Tmax_rl) -> Bus Creator/1  "Tmax_rl_Nm"
  kappa_rl/1 -> Slip Correction Left/1(kappa_rl)
  kappa_rr/1 -> Slip Correction Right/2(kappa_rr)
  Fz/1 -> Bus Selector/1
  Bus Selector/1 -> Slip Correction Left/2(Fz_rl)  "<Fz_rl>"
  Bus Selector/2 -> Slip Correction Right/1(Fz_rr)  "<Fz_rr>"
  Bus Creator/1 -> Tmax/1

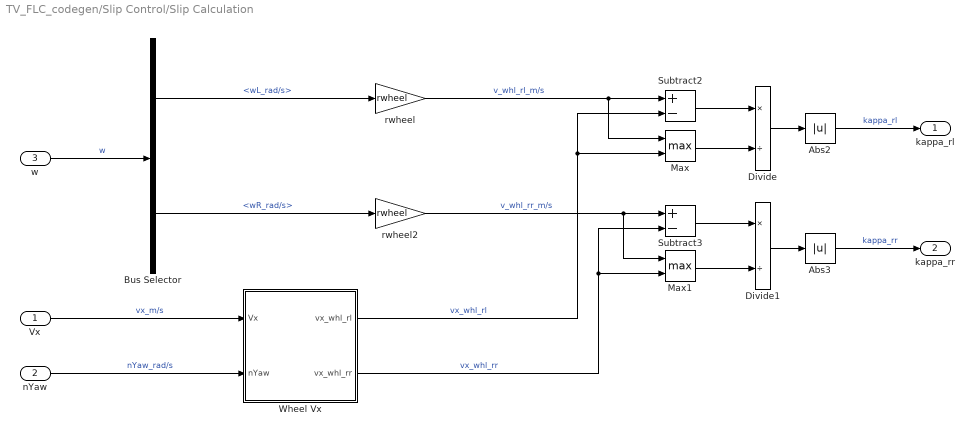
== system TV_FLC_codegen/Slip Control/Slip Calculation ==
  Vx : Inport
  nYaw : Inport  Port=2
  w : Inport  Port=3
  Abs2 : Abs  SaturateOnIntegerOverflow=off
  Abs3 : Abs  SaturateOnIntegerOverflow=off
  Bus Selector : BusSelector  OutputSignals=wL_rad/s,wR_rad/s
  Divide : Product  Inputs=*/
  Divide1 : Product  Inputs=*/
  Max : MinMax  Function=max  Inputs=2
  Max1 : MinMax  Function=max  Inputs=2
  Subtract2 : Sum  Inputs=+-
  Subtract3 : Sum  Inputs=+-
  Wheel Vx : Subsystem
  rwheel : Gain  Gain=rwheel
  rwheel2 : Gain  Gain=rwheel
  kappa_rl : Outport
  kappa_rr : Outport  Port=2
  wires:
  Bus Selector/1 -> rwheel/1  "<wL_rad/s>"
  Bus Selector/2 -> rwheel2/1  "<wR_rad/s>"
  Vx/1 -> Wheel Vx/1(Vx)  "vx_m/s"
  w/1 -> Bus Selector/1  "w"
  rwheel/1 -> Max/1, Subtract2/1  "v_whl_rl_m/s"
  rwheel2/1 -> Max1/1, Subtract3/1  "v_whl_rr_m/s"
  nYaw/1 -> Wheel Vx/2(nYaw)  "nYaw_rad/s"
  Abs3/1 -> kappa_rr/1  "kappa_rr"
  Wheel Vx/1(vx_whl_rl) -> Subtract2/2, Max/2  "vx_whl_rl"
  Abs2/1 -> kappa_rl/1  "kappa_rl"
  Subtract2/1 -> Divide/1
  Wheel Vx/2(vx_whl_rr) -> Subtract3/2, Max1/2  "vx_whl_rr"
  Subtract3/1 -> Divide1/1
  Divide/1 -> Abs2/1
  Max/1 -> Divide/2
  Divide1/1 -> Abs3/1
  Max1/1 -> Divide1/2

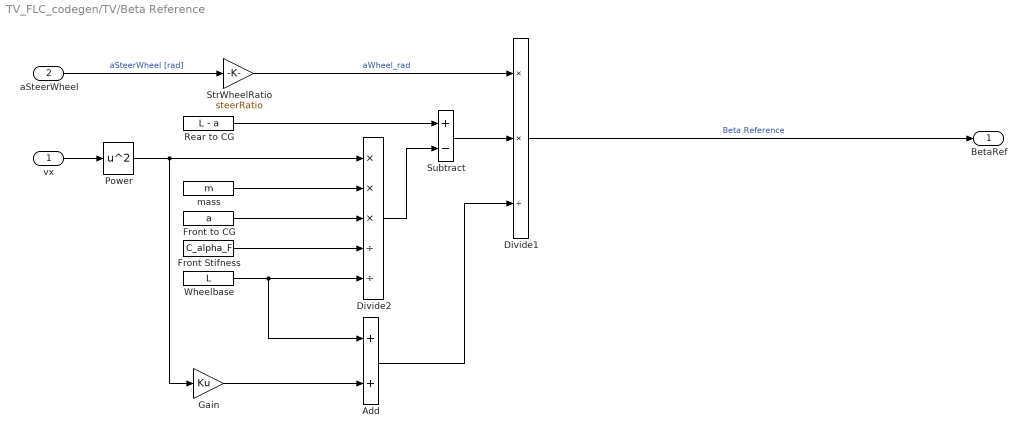
== system TV_FLC_codegen/TV/Beta Reference ==
  vx : Inport  OutDataTypeStr=single
  aSteerWheel : Inport  Port=2  OutDataTypeStr=single
  Add : Sum  OutDataTypeStr=single  AccumDataTypeStr=single
  Divide1 : Product  Inputs=**/  OutDataTypeStr=single
  Divide2 : Product  Inputs=***//  OutDataTypeStr=single
  Front Stifness : Constant  Value=C_alpha_F  OutDataTypeStr=single
  Front to CG : Constant  Value=a  OutDataTypeStr=single
  Gain : Gain  Gain=Ku  ParamDataTypeStr=single  OutDataTypeStr=single
  Power : Math  Operator=square  OutDataTypeStr=single
  Rear to CG : Constant  Value=L - a  OutDataTypeStr=single
  StrWheelRatio : Gain  Gain=steerRatio  ParamDataTypeStr=single  OutDataTypeStr=single
  Subtract : Sum  Inputs=+-  OutDataTypeStr=single  AccumDataTypeStr=single
  Wheelbase : Constant  Value=L  OutDataTypeStr=single
  mass : Constant  Value=m  OutDataTypeStr=single
  BetaRef : Outport  OutDataTypeStr=single
  wires:
  StrWheelRatio/1 -> Divide1/1  "aWheel_rad"
  Add/1 -> Divide1/3
  Gain/1 -> Add/2
  Power/1 -> Gain/1, Divide2/1
  Divide1/1 -> BetaRef/1  "Beta Reference"
  vx/1 -> Power/1
  aSteerWheel/1 -> StrWheelRatio/1  "aSteerWheel [rad]"
  Wheelbase/1 -> Add/1, Divide2/5
  Front Stifness/1 -> Divide2/4
  mass/1 -> Divide2/2
  Front to CG/1 -> Divide2/3
  Rear to CG/1 -> Subtract/1
  Divide2/1 -> Subtract/2
  Subtract/1 -> Divide1/2

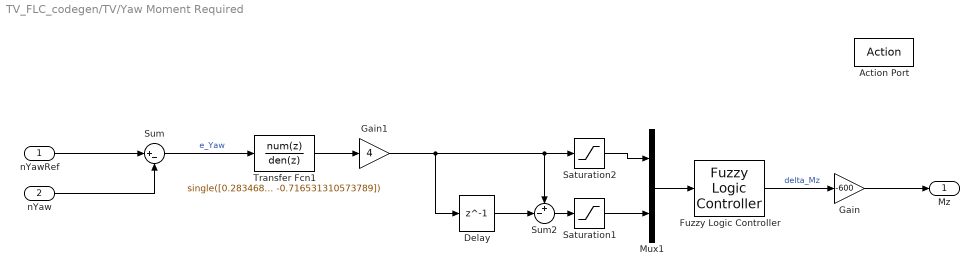
== system TV_FLC_codegen/TV/Yaw Moment Required ==
  nYawRef : Inport  OutDataTypeStr=single
  nYaw : Inport  Port=2  OutDataTypeStr=single
  Action Port : ActionPort  ActionPortLabel=case [ 1 ]:
  Delay : Delay  DelayLength=1  InputProcessing=Columns as channels (frame based)
  Fuzzy Logic Controller : fuzblock/Fuzzy Logic  Controller  FIS=FIS_1  OutputSampleNumber=200  DataType=single  UseLookupTable=off  NumBreakpoints=10  FuzzifiedInputs=off  RuleFiringStrengths=off  RuleOutputs=off  AggregatedOutputs=off  SimulateUsing=Code generation  OutOfRangeInputValueMessage=warning  NoRuleFiredMessage=warning  EmptyOutputFuzzySetMessage=warning
      link override InputConversion: OutDataTypeStr=single
  Gain : Gain  Gain=-600  ParamDataTypeStr=single  OutDataTypeStr=single
  Gain1 : Gain  Gain=4  ParamDataTypeStr=single  OutDataTypeStr=single
  Mux1 : Mux  Inputs=2
  Saturation1 : Saturate  UpperLimit=1  LowerLimit=-1  ZeroCross=off  OutDataTypeStr=single
  Saturation2 : Saturate  UpperLimit=1  LowerLimit=-1  ZeroCross=off  OutDataTypeStr=single
  Sum : Sum  Inputs=|+-  OutDataTypeStr=single  AccumDataTypeStr=single
  Sum2 : Sum  Inputs=+-|  OutDataTypeStr=single  AccumDataTypeStr=single
  Transfer Fcn1 : DiscreteTransferFcn  Numerator=single([0.283468689426211])  Denominator=single([1 -0.716531310573789])  SampleTime=0.003
  Mz : Outport  OutDataTypeStr=single
  wires:
  Gain1/1 -> Delay/1, Saturation2/1, Sum2/1
  Mux1/1 -> Fuzzy Logic Controller/1
  Sum2/1 -> Saturation1/1
  Delay/1 -> Sum2/2
  Saturation2/1 -> Mux1/1
  Saturation1/1 -> Mux1/2
  Gain/1 -> Mz/1
  Fuzzy Logic Controller/1 -> Gain/1  "delta_Mz"
  nYawRef/1 -> Sum/1
  nYaw/1 -> Sum/2
  Sum/1 -> Transfer Fcn1/1  "e_Yaw"
  Transfer Fcn1/1 -> Gain1/1

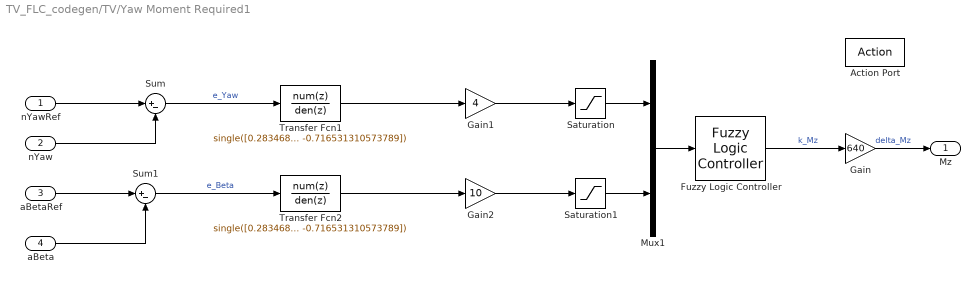
== system TV_FLC_codegen/TV/Yaw Moment Required1 ==
  nYawRef : Inport  OutDataTypeStr=single
  nYaw : Inport  Port=2  OutDataTypeStr=single
  aBetaRef : Inport  Port=3  OutDataTypeStr=single
  aBeta : Inport  Port=4  OutDataTypeStr=single
  Action Port : ActionPort  ActionPortLabel=case [ 2 ]:
  Fuzzy Logic Controller : fuzblock/Fuzzy Logic  Controller  FIS=FIS_2  OutputSampleNumber=101  DataType=single  UseLookupTable=off  NumBreakpoints=10  FuzzifiedInputs=off  RuleFiringStrengths=off  RuleOutputs=off  AggregatedOutputs=off  SimulateUsing=Code generation  OutOfRangeInputValueMessage=warning  NoRuleFiredMessage=warning  EmptyOutputFuzzySetMessage=warning
      link override InputConversion: OutDataTypeStr=single
  Gain : Gain  Gain=640  ParamDataTypeStr=single  OutDataTypeStr=single
  Gain1 : Gain  Gain=4  ParamDataTypeStr=single  OutDataTypeStr=single
  Gain2 : Gain  Gain=10  ParamDataTypeStr=single  OutDataTypeStr=single
  Mux1 : Mux  Inputs=2
  Saturation : Saturate  UpperLimit=1  LowerLimit=-1  ZeroCross=off  OutDataTypeStr=single
  Saturation1 : Saturate  UpperLimit=1  LowerLimit=-1  ZeroCross=off  OutDataTypeStr=single
  Sum : Sum  Inputs=|+-  OutDataTypeStr=single  AccumDataTypeStr=single
  Sum1 : Sum  Inputs=|+-  OutDataTypeStr=single  AccumDataTypeStr=single
  Transfer Fcn1 : DiscreteTransferFcn  Numerator=single([0.283468689426211])  Denominator=single([1 -0.716531310573789])  SampleTime=0.003
  Transfer Fcn2 : DiscreteTransferFcn  Numerator=single([0.283468689426211])  Denominator=single([1 -0.716531310573789])  SampleTime=0.003
  Mz : Outport  OutDataTypeStr=single
  wires:
  Saturation1/1 -> Mux1/2
  Saturation/1 -> Mux1/1
  aBeta/1 -> Sum1/2
  aBetaRef/1 -> Sum1/1
  nYaw/1 -> Sum/2
  nYawRef/1 -> Sum/1
  Fuzzy Logic Controller/1 -> Gain/1  "k_Mz"
  Gain/1 -> Mz/1  "delta_Mz"
  Mux1/1 -> Fuzzy Logic Controller/1
  Gain2/1 -> Saturation1/1
  Gain1/1 -> Saturation/1
  Sum/1 -> Transfer Fcn1/1  "e_Yaw"
  Transfer Fcn1/1 -> Gain1/1
  Sum1/1 -> Transfer Fcn2/1  "e_Beta"
  Transfer Fcn2/1 -> Gain2/1

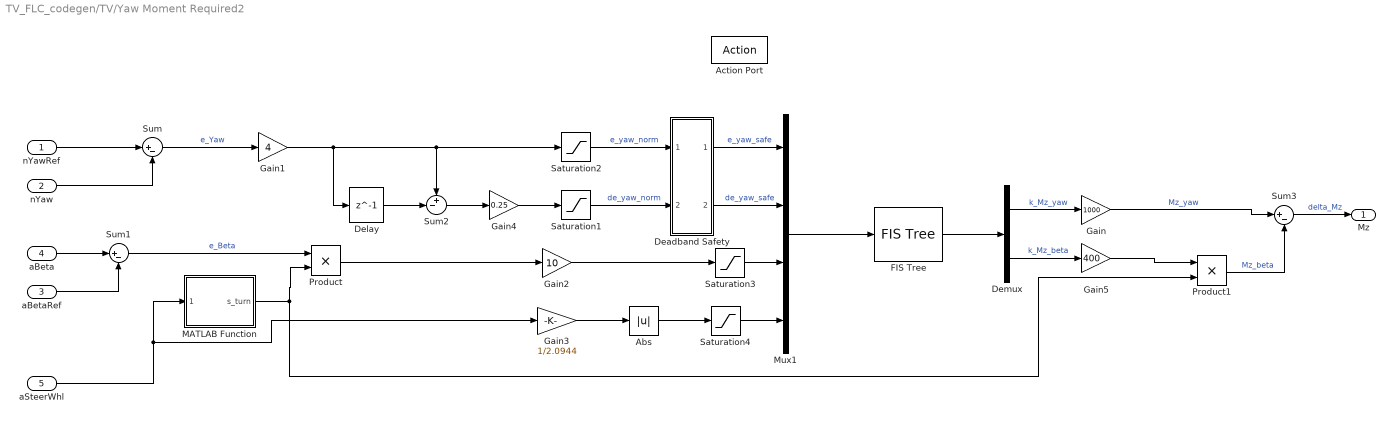
== system TV_FLC_codegen/TV/Yaw Moment Required2 ==
  nYawRef : Inport  OutDataTypeStr=single
  nYaw : Inport  Port=2  OutDataTypeStr=single
  aBetaRef : Inport  Port=3  OutDataTypeStr=single
  aBeta : Inport  Port=4  OutDataTypeStr=single
  aSteerWhl : Inport  Port=5  OutDataTypeStr=single
  Action Port : ActionPort  ActionPortLabel=case [ 3 ]:
  Abs : Abs  SaturateOnIntegerOverflow=off
  Deadband Safety : Subsystem
  Delay : Delay  DelayLength=1  InputProcessing=Columns as channels (frame based)
  Demux : Demux  Outputs=2
  FIS Tree : fuzblock/FIS Tree  FIS=FIS_3  OutputSampleNumber=101  DataType=single  SimulateUsing=Code generation  OutOfRangeInputValueMessage=warning  NoRuleFiredMessage=warning  EmptyOutputFuzzySetMessage=warning
      link override FLC Blocks/fis1/InputConversion: OutDataTypeStr=single
      link override FLC Blocks/fis2/InputConversion: OutDataTypeStr=single
      link override InputConversion: OutDataTypeStr=single
  Gain : Gain  Gain=1000  ParamDataTypeStr=single  OutDataTypeStr=single
  Gain1 : Gain  Gain=4  ParamDataTypeStr=single  OutDataTypeStr=single
  Gain2 : Gain  Gain=10  ParamDataTypeStr=single  OutDataTypeStr=single
  Gain3 : Gain  Gain=1/2.0944  ParamDataTypeStr=single  OutDataTypeStr=single
  Gain4 : Gain  Gain=0.25  ParamDataTypeStr=single  OutDataTypeStr=single
  Gain5 : Gain  Gain=400  ParamDataTypeStr=single  OutDataTypeStr=single
  MATLAB Function : MATLAB Function  TreatAsAtomicUnit=on  mask{delta_th=2}
      mask prompts: delta_th "Steering Th"
  Mux1 : Mux
  Product : Product  OutDataTypeStr=single
  Product1 : Product  OutDataTypeStr=single
  Saturation{1..4} (4 alike) : Saturate  UpperLimit=1  LowerLimit=-1  OutDataTypeStr=single
  Sum : Sum  Inputs=|+-  OutDataTypeStr=single  AccumDataTypeStr=single
  Sum1 : Sum  Inputs=|+-  OutDataTypeStr=single  AccumDataTypeStr=single
  Sum2 : Sum  Inputs=+-|  OutDataTypeStr=single  AccumDataTypeStr=single
  Sum3 : Sum  Inputs=|+-  OutDataTypeStr=single  AccumDataTypeStr=single
  Mz : Outport  OutDataTypeStr=single
  wires:
  Deadband Safety/2(de_yaw_safe) -> Mux1/2  "de_yaw_safe"
  Deadband Safety/1(e_yaw_safe) -> Mux1/1  "e_yaw_safe"
  Saturation1/1 -> Deadband Safety/2(de_yaw_norm)  "de_yaw_norm"
  Saturation2/1 -> Deadband Safety/1(e_yaw_norm)  "e_yaw_norm"
  Abs/1 -> Saturation4/1
  Product1/1 -> Sum3/2  "Mz_beta"
  Gain5/1 -> Product1/1
  Sum3/1 -> Mz/1  "delta_Mz"
  Demux/2 -> Gain5/1  "k_Mz_beta"
  Demux/1 -> Gain/1  "k_Mz_yaw"
  Product/1 -> Gain2/1
  MATLAB Function/1(s_turn) -> Product1/2, Product/2
  Gain4/1 -> Saturation1/1
  Saturation4/1 -> Mux1/4
  Saturation3/1 -> Mux1/3
  Gain3/1 -> Abs/1
  Gain2/1 -> Saturation3/1
  Gain1/1 -> Delay/1, Saturation2/1, Sum2/1
  aSteerWhl/1 -> MATLAB Function/1(delta_SW), Gain3/1
  aBetaRef/1 -> Sum1/2
  aBeta/1 -> Sum1/1
  Sum1/1 -> Product/1  "e_Beta"
  Mux1/1 -> FIS Tree/1
  Sum2/1 -> Gain4/1
  Delay/1 -> Sum2/2
  Gain/1 -> Sum3/1  "Mz_yaw"
  FIS Tree/1 -> Demux/1
  nYawRef/1 -> Sum/1
  nYaw/1 -> Sum/2
  Sum/1 -> Gain1/1  "e_Yaw"

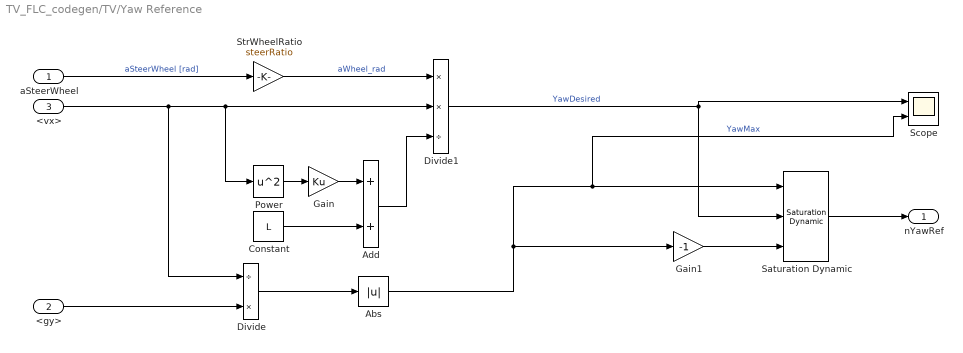
== system TV_FLC_codegen/TV/Yaw Reference ==
  aSteerWheel : Inport
  <gy> : Inport  Port=2
  <vx> : Inport  Port=3
  Abs : Abs  SaturateOnIntegerOverflow=off
  Add : Sum
  Constant : Constant  Value=L
  Divide : Product  Inputs=/*
  Divide1 : Product  Inputs=**/
  Gain : Gain  Gain=Ku
  Gain1 : Gain  Gain=-1
  Power : Math  Operator=square
  Saturation Dynamic : simulink/Discontinuities/Saturation Dynamic  OutMin=[]  OutMax=[]  OutDataTypeStr=Inherit: Same as second input  OutDataType=fixdt(1, 16)  OutScaling=2^-10  DoSatur=off
  Scope : Scope  NumInputPorts=2
      settings: ActiveDisplayYMinimum=-0.77317443098288718  ActiveDisplayYMaximum=1.3059782096862267  DataLoggingVariableName=ScopeData4
  StrWheelRatio : Gain  Gain=steerRatio
  nYawRef : Outport
  wires:
  StrWheelRatio/1 -> Divide1/1  "aWheel_rad"
  aSteerWheel/1 -> StrWheelRatio/1  "aSteerWheel [rad]"
  <vx>/1 -> Divide1/2, Power/1, Divide/1
  <gy>/1 -> Divide/2
  Divide/1 -> Abs/1
  Saturation Dynamic/1 -> nYawRef/1
  Abs/1 -> Saturation Dynamic/1, Scope/2, Gain1/1  "YawMax"
  Gain1/1 -> Saturation Dynamic/3
  Divide1/1 -> Saturation Dynamic/2, Scope/1  "YawDesired"
  Power/1 -> Gain/1
  Gain/1 -> Add/1
  Constant/1 -> Add/2
  Add/1 -> Divide1/3
